simulink model "simul"  (R2021b)
settings: Solver=VariableStepAuto  StartTime=0.0  StopTime=10.0  RelTol=1e-3
values from neighbouring files (symbols this model uses):
  K = place(A,B,P)    [q13.m]    (also in q21.m = lqr(A,B,R,Q); q8.m = [0 0 0 0])
settings Model: Creator=Arthur  LastModifiedBy=Arthur
settings DataIOCC: ExternalInput=Rref  SaveFormat=Array

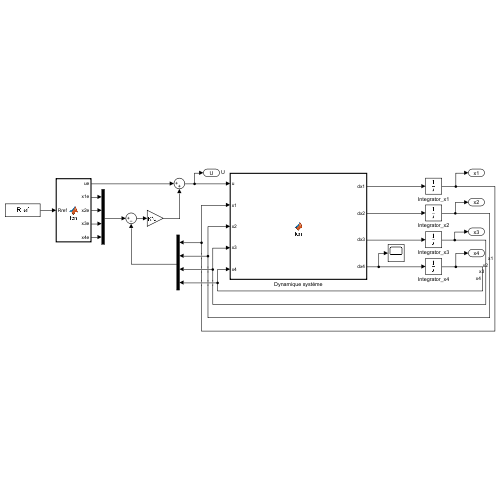
[thumbnail: Simulink's stored preview of the top-level diagram]
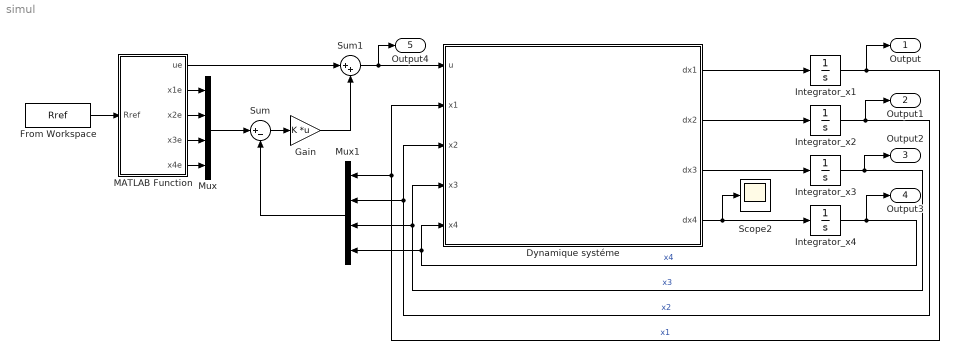
== system simul ==
  Dynamique systéme : MATLAB Function  TreatAsAtomicUnit=on
  From Workspace : FromWorkspace  VariableName=Rref  OutDataTypeStr=double  SampleTime=0.01
  Gain : Gain  Gain=K  Multiplication=Matrix(K*u)
  Integrator_x1 : Integrator  InitialCondition=0.1
  Integrator_x2 : Integrator
  Integrator_x3 : Integrator
  Integrator_x4 : Integrator
  MATLAB Function : MATLAB Function  TreatAsAtomicUnit=on
  Mux : Mux
  Mux1 : Mux
  Scope2 : Scope
  Sum : Sum  Inputs=|+-
  Sum1 : Sum  Inputs=|++
  Output : Outport
  Output1 : Outport  Port=2
  Output2 : Outport  Port=3
  Output3 : Outport  Port=4
  Output4 : Outport  Port=5  SignalName=U
  wires:
  Dynamique systéme/1(dx1) -> Integrator_x1/1
  Dynamique systéme/2(dx2) -> Integrator_x2/1
  Dynamique systéme/3(dx3) -> Integrator_x3/1
  Dynamique systéme/4(dx4) -> Scope2/1, Integrator_x4/1
  Integrator_x4/1 -> Output3/1, Mux1/4, Dynamique systéme/5(x4)  "x4"
  Integrator_x3/1 -> Mux1/3, Dynamique systéme/4(x3), Output2/1  "x3"
  Integrator_x2/1 -> Mux1/2, Dynamique systéme/3(x2), Output1/1  "x2"
  Integrator_x1/1 -> Mux1/1, Dynamique systéme/2(x1), Output/1  "x1"
  MATLAB Function/2(x1e) -> Mux/1
  MATLAB Function/3(x2e) -> Mux/2
  MATLAB Function/4(x3e) -> Mux/3
  MATLAB Function/5(x4e) -> Mux/4
  Mux/1 -> Sum/1
  Mux1/1 -> Sum/2
  Sum/1 -> Gain/1
  Sum1/1 -> Dynamique systéme/1(u), Output4/1
  MATLAB Function/1(ue) -> Sum1/1
  From Workspace/1 -> MATLAB Function/1(Rref)
  Gain/1 -> Sum1/2

== matlab function simul/MATLAB Function ==
  data: Rref input; ue output; x1e output; x2e output; x3e output; x4e output
function [ue,x1e,x2e,x3e,x4e] = fcn(Rref)
    % declaration constants
    m = 0.6; % kg
    g = 9.81; % m/s^2

    x1e = Rref;
    x2e = 0;
    x3e = 0;
    x4e = 0;
    ue = m*g*x1e;

== matlab function simul/Dynamique systéme ==
  data: u input; dx1 output; x1 input; x2 input; x3 input; x4 input; dx2 output; dx3 output; dx4 output
function [dx1,dx2,dx3,dx4] = fcn(u,x1,x2,x3,x4)
    % declaration constants
    J = 0.02; % kg.m^2
    m = 0.6; % kg
    sigma = 0.8; % adimentional
    g = 9.81; % m/s^2
    
    % dynamique
    dx1 = x2;
    dx2 = (x1*x4*x4-g*sin(x3))/(1+sigma);
    dx3 = x4;
    dx4 = (u-m*g*x1*cos(x3)-2*m*x1*x2*x4)/(J+m*x1*x1);
